simulink model "kchange"  (R2021b)
settings: Solver=VariableStepAuto  StartTime=0.0  StopTime=10.0  MaxStep=0.0005  RelTol=1e-3
settings Model: Creator=95896  LastModifiedBy=95896

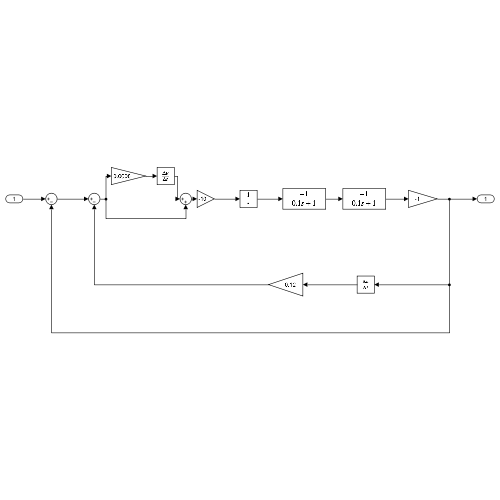
[thumbnail: Simulink's stored preview of the top-level diagram]
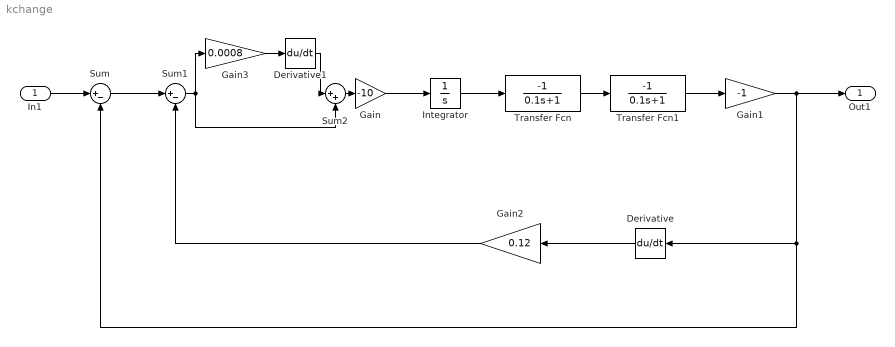
== system kchange ==
  In1 : Inport
  Derivative : Derivative
  Derivative1 : Derivative
  Gain : Gain  Gain=-10
  Gain1 : Gain  Gain=-1
  Gain2 : Gain  Gain=0.12
  Gain3 : Gain  Gain=0.0008
  Integrator : Integrator
  Sum : Sum  Inputs=|+-
  Sum1 : Sum  Inputs=|+-
  Sum2 : Sum  Inputs=|++
  Transfer Fcn : TransferFcn  Numerator=[-1]  Denominator=[0.1 1]
  Transfer Fcn1 : TransferFcn  Numerator=[-1]  Denominator=[0.1 1]
  Out1 : Outport
  wires:
  In1/1 -> Sum/1
  Sum/1 -> Sum1/1
  Sum1/1 -> Sum2/2, Gain3/1
  Gain/1 -> Integrator/1
  Integrator/1 -> Transfer Fcn/1
  Transfer Fcn/1 -> Transfer Fcn1/1
  Transfer Fcn1/1 -> Gain1/1
  Gain1/1 -> Out1/1, Derivative/1, Sum/2
  Derivative/1 -> Gain2/1
  Gain2/1 -> Sum1/2
  Gain3/1 -> Derivative1/1
  Derivative1/1 -> Sum2/1
  Sum2/1 -> Gain/1
